simulink model "untitled_restored_from_autosave"  (R2020a)
settings: Solver=VariableStepAuto  StartTime=0.0  StopTime=0.0  RelTol=1e-3
(part 1 of 2)
settings Model: Creator=KevinChan  LastModifiedBy=KevinChan

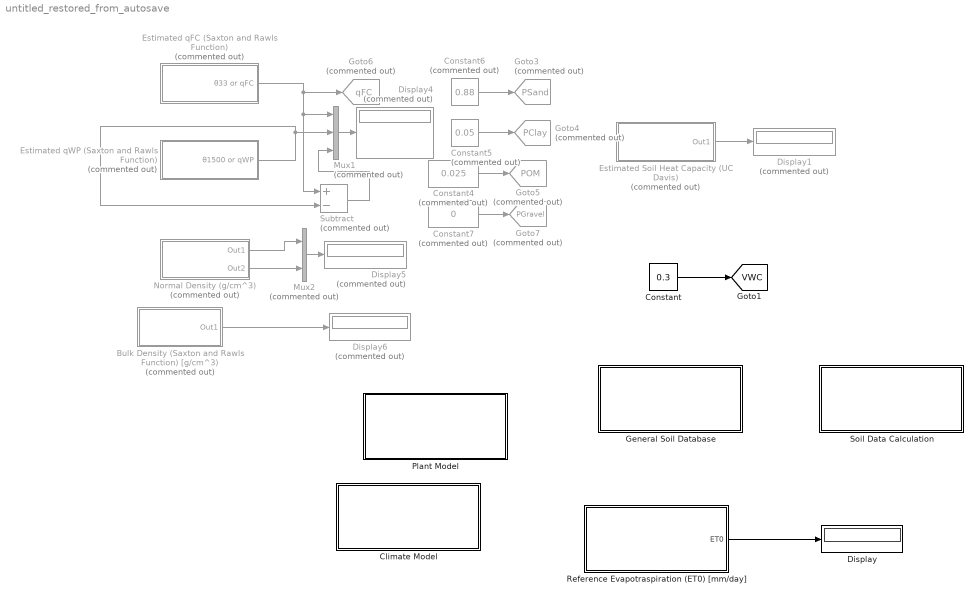
== system untitled_restored_from_autosave ==
  Bulk Density (Saxton and Rawls Function) [g/cm^3) : Subsystem  Commented=on
  Climate Model : Subsystem
  Constant : Constant  Value=0.3
  Constant4 : Constant  Commented=on  Value=0.025
  Constant5 : Constant  Commented=on  Value=0.05
  Constant6 : Constant  Commented=on  Value=0.88
  Constant7 : Constant  Commented=on  Value=0
  Display : Display
  Display{1,4..6} (4 alike) : Display  Commented=on
  Estimated Soil Heat Capacity (UC Davis) : Subsystem  Commented=on
  Estimated qFC (Saxton and Rawls Function) : Subsystem  Commented=on
  Estimated qWP (Saxton and Rawls Function) : Subsystem  Commented=on
  General Soil Database : Subsystem  mask{PGravel=5, PSand=25, PClay=30, POM=5, SM_choice=Estimated Soil Moisture Value, qFC_measured=0, qWP_measured=0, Ze_choice=Estimated, Ze_measured=0}
      mask prompts: PGravel "Percentage of Gravel"; PSand "Percentage of Sand"; PClay "Percentage of Clay"; POM "Percentage of Organic Matter (3-6% if unkown)"; SM_choice "Estimated or measured?"; qFC_measured "Field Capacity Soil Moisture (% Volume in m)"; qWP_measured "Wiliting Point Soil Moisture (% Volume in m)"; Ze_choice "Ze estimated or measured?"; Ze_measured "Enter Ze measured if selected"
      mask TypeOptions SM_choice: Estimated Soil Moisture Value | Measured Soil Moisture Value
      mask TypeOptions Ze_choice: Estimated | Measured
      mask DialogControl Container5 Prompt: Percentage of Gravel (%)
      mask DialogControl ParameterGroupVar Prompt: Percentage of Soil Content excluding Gravel (%)
      mask DialogControl Control2 Prompt: Percentage of Silt is not required
      mask DialogControl Container3 Prompt: Soil Moisture Data (more accurate if measured)
      mask DialogControl Control3 Prompt: Fill the following if you selected measured
      mask DialogControl Container8 Prompt: Ze depth of the surface soil layer that is subject to drying by way of evaporation [0.10-0.15m]
  Goto3 : Goto  Commented=on  GotoTag=PSand  TagVisibility=global
  Goto4 : Goto  Commented=on  GotoTag=PClay  TagVisibility=global
  Goto5 : Goto  Commented=on  GotoTag=POM  TagVisibility=global
  Goto6 : Goto  Commented=on  GotoTag=qFC  TagVisibility=global
  Goto7 : Goto  Commented=on  GotoTag=PGravel  TagVisibility=global
  Mux1 : Mux  Commented=on  Inputs=3
  Mux2 : Mux  Commented=on  Inputs=2
  Normal Density (g/cm^3) : Subsystem  Commented=on
  Plant Model : Subsystem
  Reference Evapotraspiration (ET0) [mm/day] : Subsystem
  Soil Data Calculation : Subsystem
  Subtract : Sum  Commented=on  Inputs=+-
  tag scope: VWC=global
  wires:
  Estimated qFC (Saxton and Rawls Function)/1(" θ33 or qFC") -> Subtract/1, Mux1/1, Goto6/1
  Constant4/1 -> Goto5/1
  Constant5/1 -> Goto4/1
  Constant6/1 -> Goto3/1
  Estimated qWP (Saxton and Rawls Function)/1(θ1500 or qWP) -> Subtract/2, Mux1/2
  Mux1/1 -> Display4/1
  Normal Density (g/cm^3)/1(Out1) -> Mux2/1
  Normal Density (g/cm^3)/2(Out2) -> Mux2/2
  Mux2/1 -> Display5/1
  Bulk Density (Saxton and Rawls Function) [g/cm^3)/1(Out1) -> Display6/1
  Constant7/1 -> Goto7/1
  Reference Evapotraspiration (ET0) [mm/day]/1(ET0) -> Display/1
  Estimated Soil Heat Capacity (UC Davis)/1(Out1) -> Display1/1
  Subtract/1 -> Mux1/3
  Constant/1 -> [VWC]

== system untitled_restored_from_autosave/Bulk Density (Saxton and Rawls Function) [g//cm^3) ==
  Add : Sum
  Constant : Constant
  Constant1 : Constant  Value=2.65
  Normal Density (g/cm^3) : Subsystem
  Product : Product
  Product1 : Product
  Subtract : Sum  Inputs=+-
  Volum Fraction of Gravel (g/cm^3) : Subsystem
  Out1 : Outport
  wires:
  Add/1 -> Out1/1
  Normal Density (g/cm^3)/1(Out1) -> Product/1, Volum Fraction of Gravel (g/cm^3)/1(In1)
  Subtract/1 -> Product/2
  Product/1 -> Add/1
  Constant/1 -> Subtract/1
  Product1/1 -> Add/2
  Constant1/1 -> Product1/2
  Volum Fraction of Gravel (g/cm^3)/1(Out1) -> Subtract/2, Product1/1

== system untitled_restored_from_autosave/Climate Model ==
  " Final Calculation for Data" : Subsystem
  " Historic Data" : Subsystem
  AI Prediction : Subsystem
  General Climate Database : Subsystem  mask{LatDeg=37, LatMin=28, Altitude=9.1, WindH=10}
      mask prompts: LatDeg "Latitude Degree"; LatMin "Latitude Minute"; Altitude "Altitude above Sea Level [m]"; WindH "Height of measurement above ground surface [m]"
      mask DialogControl ParameterGroupVar Prompt: Location
      mask DialogControl Container3 Prompt: Wind Measurement

== system untitled_restored_from_autosave/Estimated Soil Heat Capacity (UC Davis) ==
  Add : Sum
  Bulk Density (Saxton and Rawls Function) [g/cm^3) : Subsystem
  Constant : Constant  Value=837
  Constant1 : Constant  Value=4.19*10^6
  Gain : Gain  Gain=0.001
  Product : Product
  Product1 : Product
  Out1 : Outport
  wires:
  Add/1 -> Out1/1
  Constant/1 -> Product/1
  Bulk Density (Saxton and Rawls Function) [g/cm^3)/1(Out1) -> Gain/1
  Product/1 -> Add/1
  Product1/1 -> Add/2
  Constant1/1 -> Product1/1
  [VWC] -> Product1/2
  Gain/1 -> Product/2

== system untitled_restored_from_autosave/Estimated qFC (Saxton and Rawls Function) ==
  Constant : Constant  Value=1.283
  Constant1 : Constant  Value=0.015
  Constant2 : Constant  Value=0.374
  Product : Product  Inputs=3
  Product1 : Product
  Subtract : Sum  Inputs=++--
  θ33t : Subsystem
  " θ33 or qFC" : Outport
  wires:
  θ33t/1(Out1) -> Product1/1, Product/2, Product/1, Subtract/1
  Product/1 -> Subtract/2
  Constant/1 -> Product/3
  Constant1/1 -> Subtract/4
  Subtract/1 -> " θ33 or qFC"/1
  Product1/1 -> Subtract/3
  Constant2/1 -> Product1/2

== system untitled_restored_from_autosave/Estimated qWP (Saxton and Rawls Function) ==
  Constant : Constant  Value=0.14
  Constant1 : Constant  Value=0.02
  Product : Product
  Subtract : Sum  Inputs=++-
  θ1500t : Subsystem
  θ1500 or qWP : Outport
  wires:
  Subtract/1 -> θ1500 or qWP/1
  Constant/1 -> Product/2
  θ1500t/1(Out1) -> Subtract/1, Product/1
  Constant1/1 -> Subtract/3
  Product/1 -> Subtract/2

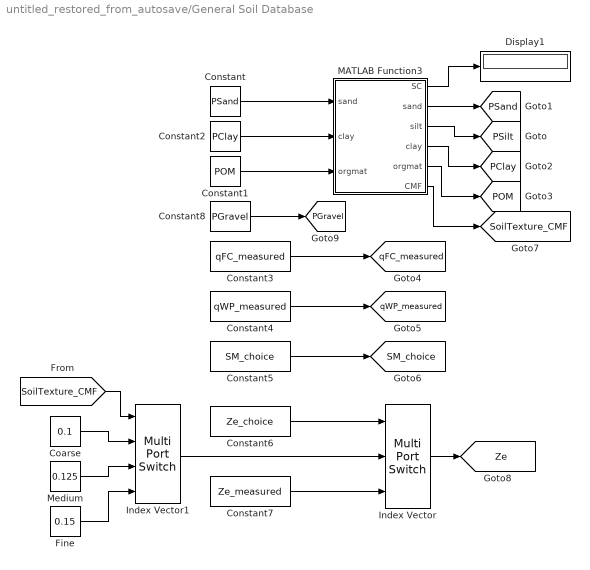
== system untitled_restored_from_autosave/General Soil Database ==
  Coarse : Constant  Value=0.1
  Constant : Constant  Value=PSand
  Constant1 : Constant  Value=POM
  Constant2 : Constant  Value=PClay
  Constant3 : Constant  Value=qFC_measured
  Constant4 : Constant  Value=qWP_measured
  Constant5 : Constant  Value=SM_choice
  Constant6 : Constant  Value=Ze_choice
  Constant7 : Constant  Value=Ze_measured
  Constant8 : Constant  Value=PGravel
  Display1 : Display
  Fine : Constant  Value=0.15
  Index Vector : MultiPortSwitch  Inputs=2
  Index Vector1 : MultiPortSwitch
  MATLAB Function3 : MATLAB Function  TreatAsAtomicUnit=on
  Medium : Constant  Value=0.125
  tag scope: PClay=global, PGravel=global, POM=global, PSand=global, PSilt=global, SM_choice=global, SoilTexture_CMF=global, Ze=global, qFC_measured=global, qWP_measured=global
  wires:
  MATLAB Function3/1(SC) -> Display1/1
  Constant2/1 -> MATLAB Function3/2("clay ")
  Constant1/1 -> MATLAB Function3/3("orgmat ")
  Constant/1 -> MATLAB Function3/1("sand ")
  MATLAB Function3/3(silt) -> [PSilt]
  Constant3/1 -> [qFC_measured]
  Constant4/1 -> [qWP_measured]
  Constant5/1 -> [SM_choice]
  MATLAB Function3/5(orgmat) -> [POM]
  MATLAB Function3/2(sand) -> [PSand]
  MATLAB Function3/4(clay) -> [PClay]
  MATLAB Function3/6(CMF) -> [SoilTexture_CMF]
  Constant6/1 -> Index Vector/1
  Constant7/1 -> Index Vector/3
  [SoilTexture_CMF] -> Index Vector1/1
  Index Vector1/1 -> Index Vector/2
  Coarse/1 -> Index Vector1/2
  Fine/1 -> Index Vector1/4
  Medium/1 -> Index Vector1/3
  Index Vector/1 -> [Ze]
  Constant8/1 -> [PGravel]

== system untitled_restored_from_autosave/Normal Density (g//cm^3) ==
  Constant : Constant  Value=2.65
  Constant1 : Constant
  Product : Product
  Saturated Moisture θS : Subsystem
  Subtract : Sum  Inputs=+-
  Out1 : Outport
  Out2 : Outport  Port=2
  wires:
  Product/1 -> Out1/1
  Constant/1 -> Product/2
  Subtract/1 -> Product/1
  Constant1/1 -> Subtract/1
  Saturated Moisture θS/1(Out1) -> Out2/1, Subtract/2

== system untitled_restored_from_autosave/Plant Model ==
  General Plant Database : Subsystem  mask{CropName=Maize, PD_Year=2020, PD_Month=11, PD_Day=28, Lini=0, Ldev=0, Lmid=0, Llate=0, inf_depth=0, interval_irr=1 day, Kc_ini=0, Kc_mid=0, Kc_end=0, MaxCropH=0, Kcb_ini=0, Kcb_mid=0, Kcb_end=0}
      mask prompts: CropName "Crop Name"; PD_Year "Year"; PD_Month "Month"; PD_Day "Day"; Lini "Initial Stage"; Ldev "Devloping Stage"; Lmid "Mid-season Stage"; Llate "Late Season Stage"; inf_depth "Average infiltration depth [mm]."; interval_irr "Interval of Irrigation (0 if unkwon)"; Kc_ini "Enter Kc ini from the Table"; Kc_mid "Enter Kc mid from the Table"; Kc_end "Enter Kc end from the Table"; MaxCropH "Enter Maximum Crop Height (h) (m) from the Table"; Kcb_ini "Enter Kcb ini from the Table"; Kcb_mid "Enter Kcb mid from the Table"; Kcb_end "Enter Kcb end from the Table"
      mask TypeOptions interval_irr: 1 day | 2 days | 4 days | 7 days | 10 days | 20 days
      mask DialogControl ParameterGroupVar Prompt: General
      mask DialogControl Control2 Prompt: Plant Date:
      mask DialogControl Container3 Prompt: Lengths of Crop Develop Stages
      mask DialogControl Control3 Prompt: Find the values in the following link with corresponding crop type and closest plant date:
      mask DialogControl Control4 Prompt: http://www.fao.org/3/x0490e/x0490e0b.htm#length%20of%20growth%20stages
      mask DialogControl Container4 Prompt: Single Crop Coefficients
      mask DialogControl Control5 Prompt: Find the values for your corresponding crop in the following table:
      mask DialogControl Control6 Prompt: http://www.fao.org/3/x0490e/x0490e0b.htm#tabulated%20kc%20values
      mask DialogControl Container5 Prompt: Dual Crop Coefficents
      mask DialogControl Control7 Prompt: Find the values for your corresponding crop in the following table:
      mask DialogControl Control8 Prompt: http://www.fao.org/3/x0490e/x0490e0c.htm#basal%20crop%20coefficient%20(kcb)
  Plant Data Calculation : Subsystem

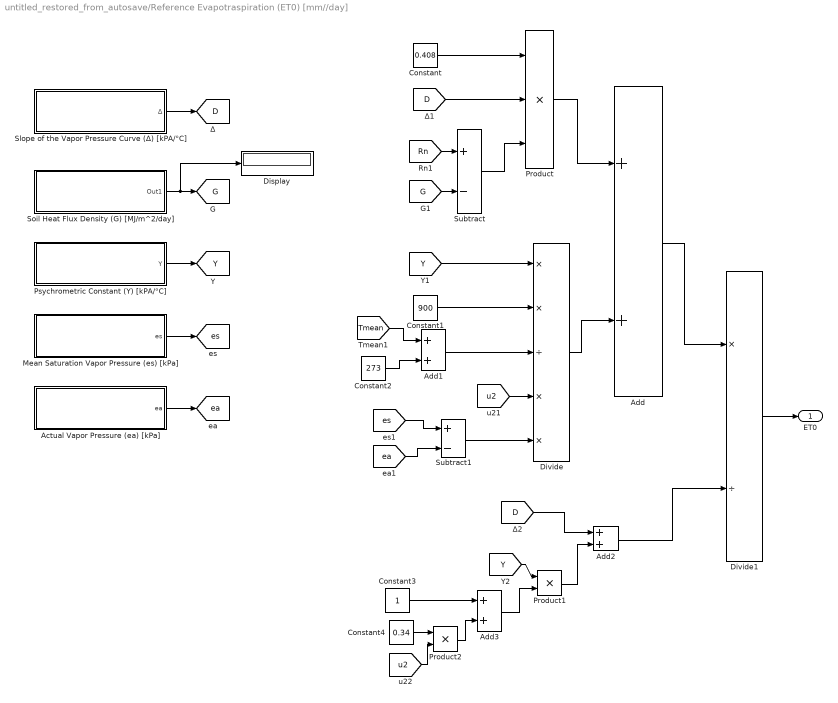
== system untitled_restored_from_autosave/Reference Evapotraspiration (ET0) [mm//day] ==
  Actual Vapor Pressure (ea) [kPa] : Subsystem  mask{ea_choice=Derived from Dewpoint Temperature, apsy_choice=0.000662 for ventilated (Asmann type) psychrometers, with an air movement of some 5 m/s}
      mask prompts: ea_choice "Select which method to derive:"; apsy_choice "Pick value for apsy:"
      mask init:
      | apsy = 0;
      | 
      | if apsy_choice == 1
      |     apsy = 0.000662;
      | elseif apsy_choice == 2
      |     apsy = 0.000800;
      | elseif apsy_choice == 3
      |     apsy = 0.001200;
      | end
      mask TypeOptions ea_choice: Derived from Dewpoint Temperature | Derived from Psyschrometirc Data | Derived from Relative Humidity Data (RHmax and RHmin) | Derived from Relative Humidity Data (RHmax only) | Derived from Relative Humidity Data (RHmean only)
      mask TypeOptions apsy_choice: 0.000662 for ventilated (Asmann type) psychrometers, with an air movement of some 5 m/s | 0.000800 for natural ventilated psychrometers (about 1 m/s) | 0.001200 for non-ventilated psychrometers installed indoors.
      mask DialogControl Control2 Prompt: There are 3 different ways to derive the actual vapor pressure. Depend on what data you have avaliable, pick the following choices. If you are picking relatitive humidity, beware of the following. When using equipment where errors in estimating RHmin can be large, or when RH data integrity are in doubt, then one should use only RHmax. In the absence of RHmax and RHmin, you can select to use RHmean.
      mask DialogControl Control3 Prompt: If you picked to use Psychrometric Data, select the folowing.
  Add{,1..3} (4 alike) : Sum
  Constant : Constant  Value=0.408
  Constant1 : Constant  Value=900
  Constant2 : Constant  Value=273
  Constant3 : Constant
  Constant4 : Constant  Value=0.34
  Display : Display
  Divide : Product  Inputs=**/**
  Divide1 : Product  Inputs=*/
  "Mean Saturation Vapor Pressure (es) [kPa] " : Subsystem
  Product : Product  Inputs=3
  Product1 : Product
  Product2 : Product
  Psychrometric Constant (Y) [kPA/°C] : Subsystem
  Slope of the Vapor Pressure Curve (∆) [kPA/°C] : Subsystem
  Soil Heat Flux Density (G) [MJ/m^2/day] : Subsystem  mask{G_choice=For day and ten-day periods}
      mask prompts: G_choice "Select Time Step:"
      mask TypeOptions G_choice: For day and ten-day periods | For long periods
      mask DialogControl Control2 Prompt: For daily or weekly periods of time, soil heat flux density is small and can be ignored. A method to find G for long period of time is here, based on the idea that the soil temperature follows air temperature.
  Subtract : Sum  Inputs=+-
  Subtract1 : Sum  Inputs=+-
  ET0 : Outport
  tag scope: D=global, G=global, Y=global, ea=global, es=global
  wires:
  Divide1/1 -> ET0/1
  Constant/1 -> Product/1
  [D] -> Product/2
  [Rn] -> Subtract/1
  [G] -> Subtract/2
  Subtract/1 -> Product/3
  Product/1 -> Add/1
  Divide/1 -> Add/2
  Constant1/1 -> Divide/2
  [Tmean] -> Add1/1
  Constant2/1 -> Add1/2
  Add1/1 -> Divide/3
  Subtract1/1 -> Divide/5
  [es] -> Subtract1/1
  [ea] -> Subtract1/2
  Add/1 -> Divide1/1
  Add2/1 -> Divide1/2
  Product1/1 -> Add2/2
  Add3/1 -> Product1/2
  Constant3/1 -> Add3/1
  Product2/1 -> Add3/2
  Slope of the Vapor Pressure Curve (∆) [kPA/°C]/1(∆) -> [D]
  [D] -> Add2/1
  Soil Heat Flux Density (G) [MJ/m^2/day]/1(Out1) -> Display/1, [G]
  Psychrometric Constant (Y) [kPA/°C]/1(Y) -> [Y]
  [Y] -> Divide/1
  [Y] -> Product1/1
  [u2] -> Divide/4
  [u2] -> Product2/2
  "Mean Saturation Vapor Pressure (es) [kPa] "/1(es) -> [es]
  Actual Vapor Pressure (ea) [kPa]/1(ea) -> [ea]
  Constant4/1 -> Product2/1

== system untitled_restored_from_autosave/Soil Data Calculation ==
  Demux : Demux  Outputs=2
  Display : Display
  Estimated Soil Heat Capacity (UC Davis) : Subsystem
  Estimated qFC (Saxton and Rawls Function) : Subsystem
  Estimated qWP (Saxton and Rawls Function) : Subsystem
  Gain : Gain  Gain=10^(-6)
  Index Vector : MultiPortSwitch  Inputs=2
  Mux : Mux  Inputs=2
  Mux1 : Mux  Inputs=2
  tag scope: cs=global, qFC=global, qWP=global
  wires:
  [SM_choice] -> Index Vector/1
  [qFC_measured] -> Mux/1
  [qWP_measured] -> Mux/2
  Mux/1 -> Index Vector/3
  Index Vector/1 -> Demux/1
  Demux/1 -> [qFC]
  Demux/2 -> [qWP]
  Mux1/1 -> Index Vector/2
  Estimated qFC (Saxton and Rawls Function)/1(" θ33 or qFC") -> Mux1/1
  Estimated qWP (Saxton and Rawls Function)/1(θ1500 or qWP) -> Mux1/2
  Estimated Soil Heat Capacity (UC Davis)/1(Out1) -> Gain/1
  Gain/1 -> Display/1, [cs]

== system untitled_restored_from_autosave/Bulk Density (Saxton and Rawls Function) [g//cm^3)/Normal Density (g//cm^3) ==
  Constant : Constant  Value=2.65
  Constant1 : Constant
  Product : Product
  Saturated Moisture θS : Subsystem
  Subtract : Sum  Inputs=+-
  Out1 : Outport
  wires:
  Product/1 -> Out1/1
  Constant/1 -> Product/2
  Subtract/1 -> Product/1
  Constant1/1 -> Subtract/1
  Saturated Moisture θS/1(Out1) -> Subtract/2

== system untitled_restored_from_autosave/Bulk Density (Saxton and Rawls Function) [g//cm^3)/Volum Fraction of Gravel (g//cm^3) ==
  In1 : Inport
  Constant : Constant  Value=2.65
  Constant1 : Constant
  Constant2 : Constant
  Divide : Product  Inputs=*/
  Divide1 : Product  Inputs=*/
  Product : Product
  Product1 : Product
  Subtract : Sum  Inputs=+-
  Subtract1 : Sum  Inputs=+-
  Out1 : Outport
  wires:
  In1/1 -> Divide/1
  [PGravel] -> Product1/1, Product/2
  Constant/1 -> Divide/2
  Divide/1 -> Subtract1/2, Product/1
  Product/1 -> Divide1/1
  Subtract/1 -> Divide1/2
  Constant1/1 -> Subtract/1
  Product1/1 -> Subtract/2
  Subtract1/1 -> Product1/2
  Constant2/1 -> Subtract1/1
  Divide1/1 -> Out1/1

== system untitled_restored_from_autosave/Climate Model/ Final Calculation for Data ==
  Atmospheric Pressure [kPa] : Subsystem
  Constant : Constant  Value=101.8
  Daily Temperature [°C] : Subsystem
  Display : Display
  Humidity : Subsystem
  Net Radiation at the Crop Surface (Rn) [MJ/m^2/day] : Subsystem
  Precipitation : Subsystem
  Wind Speed : Subsystem
  tag scope: P=global, RHmax=global, RHmean=global, RHmin=global, Rn=global, Tdew=global, Tdry=global, Tmax=global, Tmean=global, Tmin=global, Tpast=global, Tpast_t=global, Twet=global, u2=global
  wires:
  Daily Temperature [°C]/1(Tmax) -> [Tmax]
  Daily Temperature [°C]/2(Tmin) -> [Tmin]
  Daily Temperature [°C]/3(Tmean) -> [Tmean]
  Net Radiation at the Crop Surface (Rn) [MJ/m^2/day]/1(Rn) -> [Rn]
  Wind Speed/1(Out1) -> [u2]
  Daily Temperature [°C]/4(Tdew) -> [Tdew]
  Daily Temperature [°C]/5(Tdry) -> [Tdry]
  Daily Temperature [°C]/6(Twet) -> [Twet]
  Humidity/1(RHmax) -> [RHmax]
  Humidity/3(RHmean) -> [RHmean]
  Humidity/2(RHmin) -> [RHmin]
  Daily Temperature [°C]/7(Tpast) -> [Tpast]
  Daily Temperature [°C]/8(Tpast_time) -> [Tpast_t]
  Constant/1 -> [P]
  Atmospheric Pressure [kPa]/1(P) -> Display/1

== system untitled_restored_from_autosave/Climate Model/ Historic Data ==
  Humidity : Subsystem
  Precipitation : Subsystem
  Solar Radiation : Subsystem
  Temperature [°C] : Subsystem
  "Wind Speed " : Subsystem

== system untitled_restored_from_autosave/Climate Model/AI Prediction ==
  AI Solar Radiation [MJ/m^2/day] : Subsystem
  Humidity : Subsystem
  Precipitation : Subsystem
  Temperature [°C] : Subsystem
  Wind Speed [m/s] : Subsystem
  tag scope: AI_Rs=global, AI_T=global, AI_Uz=global
  wires:
  AI Solar Radiation [MJ/m^2/day]/1(AI_Rs) -> [AI_Rs]
  Wind Speed [m/s]/1(AI_Uz) -> [AI_Uz]
  Temperature [°C]/1(AI_T) -> [AI_T]

== system untitled_restored_from_autosave/Climate Model/General Climate Database ==
  Altitude : Constant  Value=Altitude
  LatDeg : Constant  Value=LatDeg
  LatMin : Constant  Value=LatMin
  WindH : Constant  Value=WindH
  tag scope: Altitude=global, LatDeg=global, LatMin=global, WindH=global
  wires:
  Altitude/1 -> [Altitude]
  LatDeg/1 -> [LatDeg]
  LatMin/1 -> [LatMin]
  WindH/1 -> [WindH]

== system untitled_restored_from_autosave/Estimated Soil Heat Capacity (UC Davis)/Bulk Density (Saxton and Rawls Function) [g//cm^3) ==
  Add : Sum
  Constant : Constant
  Constant1 : Constant  Value=2.65
  Normal Density (g/cm^3) : Subsystem
  Product : Product
  Product1 : Product
  Subtract : Sum  Inputs=+-
  Volum Fraction of Gravel (g/cm^3) : Subsystem
  Out1 : Outport
  wires:
  Add/1 -> Out1/1
  Normal Density (g/cm^3)/1(Out1) -> Product/1, Volum Fraction of Gravel (g/cm^3)/1(In1)
  Subtract/1 -> Product/2
  Product/1 -> Add/1
  Constant/1 -> Subtract/1
  Product1/1 -> Add/2
  Constant1/1 -> Product1/2
  Volum Fraction of Gravel (g/cm^3)/1(Out1) -> Subtract/2, Product1/1

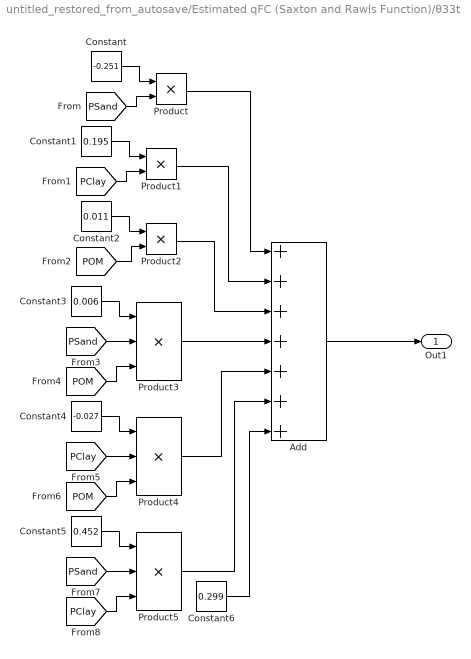
== system untitled_restored_from_autosave/Estimated qFC (Saxton and Rawls Function)/θ33t ==
  Add : Sum  Inputs=+++++++
  Constant : Constant  Value=-0.251
  Constant1 : Constant  Value=0.195
  Constant2 : Constant  Value=0.011
  Constant3 : Constant  Value=0.006
  Constant4 : Constant  Value=-0.027
  Constant5 : Constant  Value=0.452
  Constant6 : Constant  Value=0.299
  Product : Product
  Product1 : Product
  Product2 : Product
  Product3 : Product  Inputs=3
  Product4 : Product  Inputs=3
  Product5 : Product  Inputs=3
  Out1 : Outport
  wires:
  [PClay] -> Product5/3
  [PClay] -> Product1/2
  Constant4/1 -> Product4/1
  Product1/1 -> Add/2
  Constant3/1 -> Product3/1
  Product5/1 -> Add/6
  [PClay] -> Product4/2
  Product4/1 -> Add/5
  Constant6/1 -> Add/7
  Constant5/1 -> Product5/1
  [PSand] -> Product5/2
  Product/1 -> Add/1
  [PSand] -> Product/2
  Product2/1 -> Add/3
  Constant2/1 -> Product2/1
  Constant1/1 -> Product1/1
  Product3/1 -> Add/4
  Constant/1 -> Product/1
  [POM] -> Product2/2
  [PSand] -> Product3/2
  [POM] -> Product4/3
  [POM] -> Product3/3
  Add/1 -> Out1/1

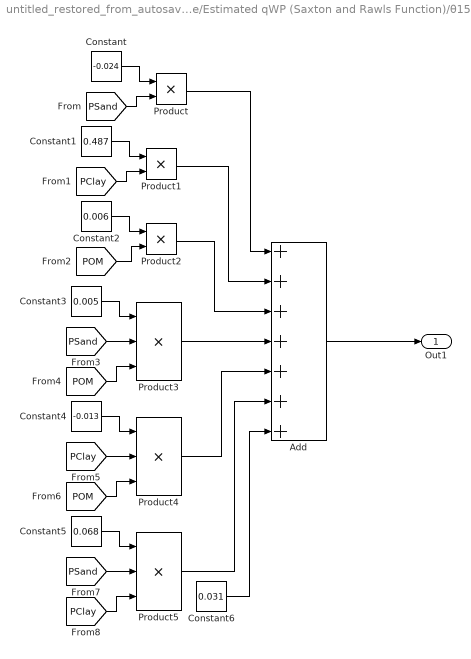
== system untitled_restored_from_autosave/Estimated qWP (Saxton and Rawls Function)/θ1500t ==
  Add : Sum  Inputs=+++++++
  Constant : Constant  Value=-0.024
  Constant1 : Constant  Value=0.487
  Constant2 : Constant  Value=0.006
  Constant3 : Constant  Value=0.005
  Constant4 : Constant  Value=-0.013
  Constant5 : Constant  Value=0.068
  Constant6 : Constant  Value=0.031
  Product : Product
  Product1 : Product
  Product2 : Product
  Product3 : Product  Inputs=3
  Product4 : Product  Inputs=3
  Product5 : Product  Inputs=3
  Out1 : Outport
  wires:
  [PClay] -> Product5/3
  [PClay] -> Product1/2
  Constant4/1 -> Product4/1
  Product1/1 -> Add/2
  Constant3/1 -> Product3/1
  Product5/1 -> Add/6
  [PClay] -> Product4/2
  Product4/1 -> Add/5
  Constant6/1 -> Add/7
  Constant5/1 -> Product5/1
  [PSand] -> Product5/2
  Product/1 -> Add/1
  [PSand] -> Product/2
  Product2/1 -> Add/3
  Constant2/1 -> Product2/1
  Constant1/1 -> Product1/1
  Product3/1 -> Add/4
  Constant/1 -> Product/1
  [POM] -> Product2/2
  [PSand] -> Product3/2
  [POM] -> Product4/3
  [POM] -> Product3/3
  Add/1 -> Out1/1

== system untitled_restored_from_autosave/Normal Density (g//cm^3)/Saturated Moisture θS ==
  Constant : Constant  Value=0.097
  Constant1 : Constant  Value=0.043
  Product : Product
  Subtract : Sum  Inputs=++-+
  θ(S-33) : Subsystem
  Out1 : Outport
  wires:
  Subtract/1 -> Out1/1
  [qFC] -> Subtract/1
  Product/1 -> Subtract/3
  Constant/1 -> Product/1
  [PSand] -> Product/2
  Constant1/1 -> Subtract/4
  θ(S-33)/1(Out1) -> Subtract/2

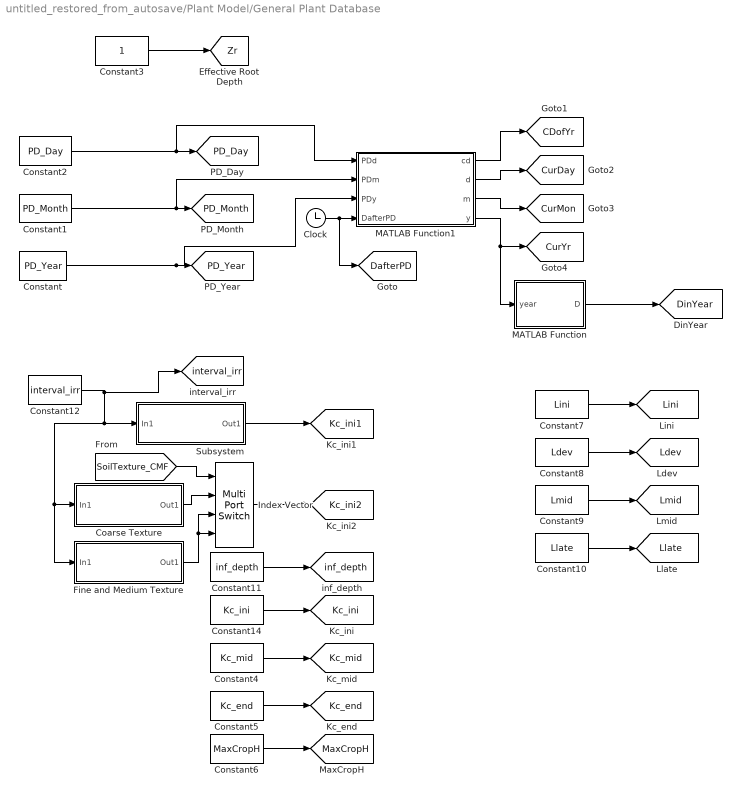
== system untitled_restored_from_autosave/Plant Model/General Plant Database ==
  Clock : Clock
  Coarse Texture : Subsystem
  Constant : Constant  Value=PD_Year
  Constant1 : Constant  Value=PD_Month
  Constant10 : Constant  Value=Llate
  Constant11 : Constant  Value=inf_depth
  Constant12 : Constant  Value=interval_irr
  Constant14 : Constant  Value=Kc_ini
  Constant2 : Constant  Value=PD_Day
  Constant3 : Constant
  Constant4 : Constant  Value=Kc_mid
  Constant5 : Constant  Value=Kc_end
  Constant6 : Constant  Value=MaxCropH
  Constant7 : Constant  Value=Lini
  Constant8 : Constant  Value=Ldev
  Constant9 : Constant  Value=Lmid
  Fine and Medium Texture : Subsystem
  Index Vector : MultiPortSwitch
  MATLAB Function : MATLAB Function  TreatAsAtomicUnit=on
  MATLAB Function1 : MATLAB Function  TreatAsAtomicUnit=on
  Subsystem : Subsystem
  tag scope: CDofYr=global, CurDay=global, CurMon=global, CurYr=global, DafterPD=global, DinYear=global, Kc_end=global, Kc_ini1=global, Kc_ini2=global, Kc_ini=global, Kc_mid=global, Ldev=global, Lini=global, Llate=global, Lmid=global, MaxCropH=global, PD_Day=global, PD_Month=global, PD_Year=global, Zr=global, inf_depth=global, interval_irr=global
  wires:
  Constant/1 -> MATLAB Function1/3(PDy), [PD_Year]
  Constant1/1 -> MATLAB Function1/2(PDm), [PD_Month]
  Constant2/1 -> MATLAB Function1/1(PDd), [PD_Day]
  MATLAB Function/1(D) -> [DinYear]
  Constant4/1 -> [Kc_mid]
  Constant5/1 -> [Kc_end]
  Constant6/1 -> [MaxCropH]
  Constant9/1 -> [Lmid]
  Constant8/1 -> [Ldev]
  Constant7/1 -> [Lini]
  Constant10/1 -> [Llate]
  Constant11/1 -> [inf_depth]
  [SoilTexture_CMF] -> Index Vector/1
  Index Vector/1 -> [Kc_ini2]
  Constant12/1 -> [interval_irr], Fine and Medium Texture/1(In1), Coarse Texture/1(In1), Subsystem/1(In1)
  Subsystem/1(Out1) -> [Kc_ini1]
  Coarse Texture/1(Out1) -> Index Vector/2
  Constant14/1 -> [Kc_ini]
  Clock/1 -> MATLAB Function1/4(DafterPD), [DafterPD]
  MATLAB Function1/1(cd) -> [CDofYr]
  MATLAB Function1/2(d) -> [CurDay]
  MATLAB Function1/3(m) -> [CurMon]
  MATLAB Function1/4(y) -> MATLAB Function/1(year), [CurYr]
  Fine and Medium Texture/1(Out1) -> Index Vector/3, Index Vector/4
  Constant3/1 -> [Zr]

== system untitled_restored_from_autosave/Plant Model/Plant Data Calculation ==
  MATLAB Function : MATLAB Function  TreatAsAtomicUnit=on
  tag scope: Ps=global
  wires:
  MATLAB Function/1(stage) -> [Ps]
  [DafterPD] -> MATLAB Function/1(d)
  [Lini] -> MATLAB Function/2(Lini)
  [Ldev] -> MATLAB Function/3(Ldev)
  [Lmid] -> MATLAB Function/4(Lmid)
  [Llate] -> MATLAB Function/5(Llate)

== system untitled_restored_from_autosave/Reference Evapotraspiration (ET0) [mm//day]/Actual Vapor Pressure (ea) [kPa] ==
  Constant : Constant  Value=ea_choice
  Derived from Dewpoint Temperature : Subsystem
  Derived from Psychrometric Data : Subsystem
  Derived from RHmax & RHmin : Subsystem
  Derived from RHmax only : Subsystem
  Derived from RHmean only : Subsystem
  Index Vector : MultiPortSwitch  Inputs=5
  ea : Outport
  wires:
  Derived from Dewpoint Temperature/1(Out1) -> Index Vector/2
  Index Vector/1 -> ea/1
  Constant/1 -> Index Vector/1
  Derived from Psychrometric Data/1(Out1) -> Index Vector/3
  Derived from RHmean only/1(Out1) -> Index Vector/6
  Derived from RHmax only/1(Out1) -> Index Vector/5
  Derived from RHmax & RHmin/1(Out1) -> Index Vector/4

== system untitled_restored_from_autosave/Reference Evapotraspiration (ET0) [mm//day]/Mean Saturation Vapor Pressure (es) [kPa]  ==
  Add2 : Sum
  Constant6 : Constant  Value=2
  Divide2 : Product  Inputs=*/
  Saturation Vapor Pressure (eo) : Subsystem
  Saturation Vapor Pressure (eo) 2 : Subsystem
  es : Outport
  wires:
  Add2/1 -> Divide2/1
  Divide2/1 -> es/1
  Constant6/1 -> Divide2/2
  [Tmax] -> Saturation Vapor Pressure (eo)/1(In1)
  Saturation Vapor Pressure (eo)/1(Out1) -> Add2/1
  [Tmin] -> Saturation Vapor Pressure (eo) 2/1(In1)
  Saturation Vapor Pressure (eo) 2/1(Out1) -> Add2/2

== system untitled_restored_from_autosave/Reference Evapotraspiration (ET0) [mm//day]/Psychrometric Constant (Y) [kPA//°C] ==
  Divide : Product  Inputs=**//
  Latent Heat of Vaporization (l) [MJ/kg] : Subsystem
  Ratio Molecular Weight of Water Vapour/Dry Air (e) : Constant  Value=0.622
  "Specific Heat at Constant Pressure (cp) [MJ/kg/°C] " : Constant  Value=0.001013
  Y : Outport
  wires:
  Divide/1 -> Y/1
  "Specific Heat at Constant Pressure (cp) [MJ/kg/°C] "/1 -> Divide/1
  Latent Heat of Vaporization (l) [MJ/kg]/1(l) -> Divide/4
  [P] -> Divide/2
  Ratio Molecular Weight of Water Vapour/Dry Air (e)/1 -> Divide/3

== system untitled_restored_from_autosave/Reference Evapotraspiration (ET0) [mm//day]/Slope of the Vapor Pressure Curve (∆) [kPA//°C] ==
  Add : Sum
  Constant : Constant  Value=4098
  Constant1 : Constant  Value=0.6108
  Constant2 : Constant  Value=17.27
  Constant3 : Constant  Value=237.3
  Divide : Product  Inputs=***//
  Divide1 : Product  Inputs=**/
  Math Function : Math  SaturateOnIntegerOverflow=on
  ∆ : Outport
  wires:
  Divide/1 -> ∆/1
  Constant/1 -> Divide/1
  Constant1/1 -> Divide/2
  Math Function/1 -> Divide/3
  Divide1/1 -> Math Function/1
  [Tmean] -> Add/1, Divide1/2
  Constant2/1 -> Divide1/1
  Add/1 -> Divide/5, Divide/4, Divide1/3
  Constant3/1 -> Add/2

== system untitled_restored_from_autosave/Reference Evapotraspiration (ET0) [mm//day]/Soil Heat Flux Density (G) [MJ//m^2//day] ==
  Constant : Constant  Value=G_choice
  For day and ten-day peroids : Constant  Value=0
  Index Vector : MultiPortSwitch  Inputs=2
  Long Time Steps : Subsystem
  Out1 : Outport
  wires:
  Long Time Steps/1(Out1) -> Index Vector/3
  For day and ten-day peroids/1 -> Index Vector/2
  Constant/1 -> Index Vector/1
  Index Vector/1 -> Out1/1

== system untitled_restored_from_autosave/Soil Data Calculation/Estimated Soil Heat Capacity (UC Davis) ==
  Add : Sum
  Bulk Density (Saxton and Rawls Function) [g/cm^3) : Subsystem
  Constant : Constant  Value=837
  Constant1 : Constant  Value=4.19*10^6
  Gain : Gain  Gain=0.001
  Product : Product
  Product1 : Product
  Out1 : Outport
  wires:
  Add/1 -> Out1/1
  Constant/1 -> Product/1
  Bulk Density (Saxton and Rawls Function) [g/cm^3)/1(Out1) -> Gain/1
  Product/1 -> Add/1
  Product1/1 -> Add/2
  Constant1/1 -> Product1/1
  [VWC] -> Product1/2
  Gain/1 -> Product/2

== system untitled_restored_from_autosave/Soil Data Calculation/Estimated qFC (Saxton and Rawls Function) ==
  Constant : Constant  Value=1.283
  Constant1 : Constant  Value=0.015
  Constant2 : Constant  Value=0.374
  Product : Product  Inputs=3
  Product1 : Product
  Subtract : Sum  Inputs=++--
  θ33t : Subsystem
  " θ33 or qFC" : Outport
  wires:
  θ33t/1(Out1) -> Product1/1, Product/2, Product/1, Subtract/1
  Product/1 -> Subtract/2
  Constant/1 -> Product/3
  Constant1/1 -> Subtract/4
  Subtract/1 -> " θ33 or qFC"/1
  Product1/1 -> Subtract/3
  Constant2/1 -> Product1/2

== system untitled_restored_from_autosave/Soil Data Calculation/Estimated qWP (Saxton and Rawls Function) ==
  Constant : Constant  Value=0.14
  Constant1 : Constant  Value=0.02
  Product : Product
  Subtract : Sum  Inputs=++-
  θ1500t : Subsystem
  θ1500 or qWP : Outport
  wires:
  Subtract/1 -> θ1500 or qWP/1
  Constant/1 -> Product/2
  θ1500t/1(Out1) -> Subtract/1, Product/1
  Constant1/1 -> Subtract/3
  Product/1 -> Subtract/2

== system untitled_restored_from_autosave/Bulk Density (Saxton and Rawls Function) [g//cm^3)/Normal Density (g//cm^3)/Saturated Moisture θS ==
  Constant : Constant  Value=0.097
  Constant1 : Constant  Value=0.043
  Product : Product
  Subtract : Sum  Inputs=++-+
  θ(S-33) : Subsystem
  Out1 : Outport
  wires:
  Subtract/1 -> Out1/1
  [qFC] -> Subtract/1
  Product/1 -> Subtract/3
  Constant/1 -> Product/1
  [PSand] -> Product/2
  Constant1/1 -> Subtract/4
  θ(S-33)/1(Out1) -> Subtract/2

== system untitled_restored_from_autosave/Climate Model/ Final Calculation for Data/Atmospheric Pressure [kPa] ==
  Constant : Constant  Value=101.3
  Constant1 : Constant  Value=5.26
  Constant2 : Constant  Value=293
  Constant3 : Constant  Value=0.0065
  Constant5 : Constant  Value=293
  Divide : Product  Inputs=*/
  Math Function : Math  Operator=pow  SaturateOnIntegerOverflow=on
  Product : Product
  Product1 : Product
  Subtract : Sum  Inputs=+-
  P : Outport
  wires:
  Product/1 -> P/1
  Constant/1 -> Product/1
  Math Function/1 -> Product/2
  Constant1/1 -> Math Function/2
  Divide/1 -> Math Function/1
  Subtract/1 -> Divide/1
  Constant2/1 -> Subtract/1
  Product1/1 -> Subtract/2
  Constant3/1 -> Product1/1
  [Altitude] -> Product1/2
  Constant5/1 -> Divide/2

== system untitled_restored_from_autosave/Climate Model/ Final Calculation for Data/Daily Temperature [°C] ==
  Constant : Constant  Value=14
  Constant1 : Constant  Value=8.7
  Constant2 : Constant  Value=11.1
  Constant3 : Constant  Value=10
  Constant4 : Constant  Value=10
  Constant5 : Constant
  Mean Air Temperature at 2m height (Tmean) [°C] : Subsystem
  Tmax : Outport
  Tmin : Outport  Port=2
  Tmean : Outport  Port=3
  Tdew : Outport  Port=4
  Tdry : Outport  Port=5
  Twet : Outport  Port=6
  Tpast : Outport  Port=7
  Tpast_time : Outport  Port=8
  wires:
  Mean Air Temperature at 2m height (Tmean) [°C]/1(Out1) -> Tmean/1
  Constant/1 -> Tmax/1
  Constant1/1 -> Tmin/1
  Constant2/1 -> Mean Air Temperature at 2m height (Tmean) [°C]/1(In1)
  Constant3/1 -> Tdew/1
  Constant4/1 -> Tpast/1
  Constant5/1 -> Tpast_time/1

== system untitled_restored_from_autosave/Climate Model/ Final Calculation for Data/Humidity ==
  Constant : Constant  Value=96
  Constant1 : Constant  Value=79
  Constant2 : Constant  Value=92.2
  RHmax : Outport
  RHmin : Outport  Port=2
  RHmean : Outport  Port=3
  wires:
  Constant/1 -> RHmax/1
  Constant1/1 -> RHmin/1
  Constant2/1 -> RHmean/1

== system untitled_restored_from_autosave/Climate Model/ Final Calculation for Data/Net Radiation at the Crop Surface (Rn) [MJ//m^2//day] ==
  Clear-Sky Solar Radiation (Rso) [MJ/m^2/day] : Subsystem
  Extraterrestrial Radiation (Ra) [MJ/m^2/day] : Subsystem
  Net Longwave Radiation (Rnl) [MJ/m^2/day] : Subsystem
  Net Solar/Shortwave Radiation (Rns) [MJ/m^2/day] : Subsystem
  Solar Radiation (Rs) [MJ/m^2/day] : Subsystem  mask{Ac_Rs=AI Predicted Solar Radiation}
      mask prompts: Ac_Rs "How to calculate Solar Radiation? (Most to Least Accurate)"
      mask TypeOptions Ac_Rs: AI Predicted Solar Radiation | Angstrom Formula if AI_Rs not avaliable | Hargreaves Formula if AI_Rs and hour of daylight is not available
  Subtract : Sum  Inputs=+-
  Rn : Outport
  tag scope: Ra=global, Rs=global, Rso=global
  wires:
  Subtract/1 -> Rn/1
  Net Solar/Shortwave Radiation (Rns) [MJ/m^2/day]/1(Out1) -> Subtract/1
  Net Longwave Radiation (Rnl) [MJ/m^2/day]/1(Rnl) -> Subtract/2
  Solar Radiation (Rs) [MJ/m^2/day]/1(Rs) -> [Rs]
  Extraterrestrial Radiation (Ra) [MJ/m^2/day]/1(Ra) -> [Ra]
  [CDofYr] -> Extraterrestrial Radiation (Ra) [MJ/m^2/day]/1(J)
  Clear-Sky Solar Radiation (Rso) [MJ/m^2/day]/1(Rso) -> [Rso]

== system untitled_restored_from_autosave/Climate Model/ Final Calculation for Data/Precipitation ==

== system untitled_restored_from_autosave/Climate Model/ Final Calculation for Data/Wind Speed ==
  Constant : Constant  Value=2.7
  Wind Speed measured at 2m height (u2) [m/s] : Subsystem
  Out1 : Outport
  wires:
  Wind Speed measured at 2m height (u2) [m/s]/1(u2) -> Out1/1
  [WindH] -> Wind Speed measured at 2m height (u2) [m/s]/2(z)
  Constant/1 -> Wind Speed measured at 2m height (u2) [m/s]/1(uz)

== system untitled_restored_from_autosave/Climate Model/ Historic Data/Humidity ==

== system untitled_restored_from_autosave/Climate Model/ Historic Data/Precipitation ==

== system untitled_restored_from_autosave/Climate Model/ Historic Data/Solar Radiation ==

== system untitled_restored_from_autosave/Climate Model/ Historic Data/Temperature [°C] ==

== system untitled_restored_from_autosave/Climate Model/ Historic Data/Wind Speed  ==

== system untitled_restored_from_autosave/Climate Model/AI Prediction/AI Solar Radiation [MJ//m^2//day] ==
  AI_Rs : Outport

== system untitled_restored_from_autosave/Climate Model/AI Prediction/Humidity ==

== system untitled_restored_from_autosave/Climate Model/AI Prediction/Precipitation ==

== system untitled_restored_from_autosave/Climate Model/AI Prediction/Temperature [°C] ==
  AI_T : Outport

== system untitled_restored_from_autosave/Climate Model/AI Prediction/Wind Speed [m//s] ==
  AI_Uz : Outport

== system untitled_restored_from_autosave/Estimated Soil Heat Capacity (UC Davis)/Bulk Density (Saxton and Rawls Function) [g//cm^3)/Normal Density (g//cm^3) ==
  Constant : Constant  Value=2.65
  Constant1 : Constant
  Product : Product
  Saturated Moisture θS : Subsystem
  Subtract : Sum  Inputs=+-
  Out1 : Outport
  wires:
  Product/1 -> Out1/1
  Constant/1 -> Product/2
  Subtract/1 -> Product/1
  Constant1/1 -> Subtract/1
  Saturated Moisture θS/1(Out1) -> Subtract/2

== system untitled_restored_from_autosave/Estimated Soil Heat Capacity (UC Davis)/Bulk Density (Saxton and Rawls Function) [g//cm^3)/Volum Fraction of Gravel (g//cm^3) ==
  In1 : Inport
  Constant : Constant  Value=2.65
  Constant1 : Constant
  Constant2 : Constant
  Divide : Product  Inputs=*/
  Divide1 : Product  Inputs=*/
  Product : Product
  Product1 : Product
  Subtract : Sum  Inputs=+-
  Subtract1 : Sum  Inputs=+-
  Out1 : Outport
  wires:
  In1/1 -> Divide/1
  [PGravel] -> Product1/1, Product/2
  Constant/1 -> Divide/2
  Divide/1 -> Subtract1/2, Product/1
  Product/1 -> Divide1/1
  Subtract/1 -> Divide1/2
  Constant1/1 -> Subtract/1
  Product1/1 -> Subtract/2
  Subtract1/1 -> Product1/2
  Constant2/1 -> Subtract1/1
  Divide1/1 -> Out1/1

== system untitled_restored_from_autosave/Normal Density (g//cm^3)/Saturated Moisture θS/θ(S-33) ==
  Constant : Constant  Value=0.636
  Constant1 : Constant  Value=0.107
  Product : Product
  Subtract : Sum  Inputs=++-
  θ(S-33)t : Subsystem
  Out1 : Outport
  wires:
  θ(S-33)t/1(Out1) -> Product/1, Subtract/1
  Product/1 -> Subtract/2
  Constant/1 -> Product/2
  Constant1/1 -> Subtract/3
  Subtract/1 -> Out1/1

== system untitled_restored_from_autosave/Plant Model/General Plant Database/Coarse Texture ==
  In1 : Inport
  2-D Lookup Table : Lookup_n-D  BreakpointsForDimension1=[0 1 2 3 4 5 6 7 8 9 10 11 12]  BreakpointsForDimension2=[1 2 3 4 5 6]  Table=|  InternalRulePriority=Speed  RndMeth=Simplest  InputSameDT=on
      | [1.15 1.15 1.15 1.15 1.15 1.15;
      | 1.15 1.15 1.15 1 0.7 0.35;
      | 1.15 1.15 1.05 0.7 0.5 0.25;
      | 1.15 1.15 0.875 0.575 0.4 0.2;
      | 1.15 1.075 0.775 0.425 0.35 0.175;
      | 1.15 1 0.65 0.4 0.28 0.15;
      | 1.13 0.94 0.575 0.35 0.25 0.125;
      | 1.1 0.86 0.52 0.3 0.21 0.1;
      | 1.075 0.8 0.45 0.27 0.18 0.08;
      | 1.05 0.73 0.41 0.23 0.16 0.07;
      | 1.01 0.675 0.375 0.21 0.14 0.06;
      | 0.975 0.63 0.34 0.19 0.13 0.055;
      | 0.925 0.6 0.31 0.175 0.12 0.05]
  Round : Rounding  Operator=round
  Out1 : Outport
  wires:
  [ET0] -> Round/1
  2-D Lookup Table/1 -> Out1/1
  In1/1 -> 2-D Lookup Table/2
  Round/1 -> 2-D Lookup Table/1

== system untitled_restored_from_autosave/Plant Model/General Plant Database/Fine and Medium Texture ==
  In1 : Inport
  2-D Lookup Table : Lookup_n-D  BreakpointsForDimension1=[0 1 2 3 4 5 6 7 8 9 10 11 12]  BreakpointsForDimension2=[1 2 3 4 5 6]  Table=|  InternalRulePriority=Speed  RndMeth=Simplest  InputSameDT=on
      | [1.15 1.15 1.15 1.15 1.15 1.15;
      | 1.15 1.15 1.15 1.15 1.15 0.65;
      | 1.15 1.15 1.15 1.125 0.85 0.45;
      | 1.15 1.15 1.1 0.87 0.7 0.38;
      | 1.15 1.15 1.025 0.7 0.6 0.325;
      | 1.15 1.125 0.95 0.65 0.5 0.275;
      | 1.15 1.1 0.875 0.6 0.45 0.225;
      | 1.15 1.06 0.81 0.54 0.4 0.2;
      | 1.15 1.025 0.73 0.48 0.35 0.175;
      | 1.14 0.98 0.675 0.43 0.3 0.15;
      | 1.125 0.94 0.63 0.39 0.275 0.125;
      | 1.1 0.9 0.59 0.35 0.25 0.11;
      | 1.08 0.85 0.55 0.31 0.225 0.1]
  Round : Rounding  Operator=round
  Out1 : Outport
  wires:
  2-D Lookup Table/1 -> Out1/1
  [ET0] -> Round/1
  In1/1 -> 2-D Lookup Table/2
  Round/1 -> 2-D Lookup Table/1

== system untitled_restored_from_autosave/Plant Model/General Plant Database/Subsystem ==
  In1 : Inport
  2-D Lookup Table : Lookup_n-D  BreakpointsForDimension1=[0 1 2 3 4 5 6 7 8 9 10 11 12]  BreakpointsForDimension2=[1 2 3 4 5 6]  Table=|  InternalRulePriority=Speed  RndMeth=Simplest  InputSameDT=on
      | [1.15 1.15 1.15 1.15 1.15 1.15; 
      | 1.15 1.15 1.15 1.15 0.9 0.5; 
      | 1.15 1.15 1 0.675 0.5 0.25;
      | 1.15 1.05 0.7 0.475 0.325 0.175;
      | 1.1 0.9 0.6 0.35 0.25 0.125;
      | 1.05 0.775 0.475 0.275 0.2 0.1;
      | 0.95 0.7 0.41 0.225 0.175 0.08;
      | 0.9 0.625 0.35 0.21 0.15 0.07;
      | 0.875 0.575 0.3 0.18 0.125 0.06;
      | 0.825 0.525 0.275 0.16 0.11 0.05;
      | 0.775 0.475 0.25 0.14 0.1 0.045;
      | 0.725 0.425 0.225 0.125 0.09 0.04;
      | 0.7 0.4 0.2 0.11 0.08 0.04]
  Round : Rounding  Operator=round
  Out1 : Outport
  wires:
  In1/1 -> 2-D Lookup Table/2
  2-D Lookup Table/1 -> Out1/1
  [ET0] -> Round/1
  Round/1 -> 2-D Lookup Table/1

== system untitled_restored_from_autosave/Reference Evapotraspiration (ET0) [mm//day]/Actual Vapor Pressure (ea) [kPa]/Derived from Dewpoint Temperature ==
  Saturation Vapor Pressure (eo) : Subsystem
  Out1 : Outport
  wires:
  [Tdew] -> Saturation Vapor Pressure (eo)/1(In1)
  Saturation Vapor Pressure (eo)/1(Out1) -> Out1/1

== system untitled_restored_from_autosave/Reference Evapotraspiration (ET0) [mm//day]/Actual Vapor Pressure (ea) [kPa]/Derived from Psychrometric Data ==
  Constant : Constant  Value=apsy
  Product : Product
  Product1 : Product
  Saturation Vapor Pressure (eo) : Subsystem
  Subtract : Sum  Inputs=+-
  Subtract1 : Sum  Inputs=+-
  Out1 : Outport
  wires:
  Subtract/1 -> Out1/1
  Saturation Vapor Pressure (eo)/1(Out1) -> Subtract/1
  [Twet] -> Subtract1/2, Saturation Vapor Pressure (eo)/1(In1)
  [Tdry] -> Subtract1/1
  Subtract1/1 -> Product/1
  Product/1 -> Subtract/2
  Product1/1 -> Product/2
  [P] -> Product1/2
  Constant/1 -> Product1/1

== system untitled_restored_from_autosave/Reference Evapotraspiration (ET0) [mm//day]/Actual Vapor Pressure (ea) [kPa]/Derived from RHmax & RHmin ==
  Add : Sum
  Constant : Constant  Value=100
  Constant1 : Constant  Value=2
  Constant2 : Constant  Value=100
  Divide : Product  Inputs=**/
  Divide1 : Product  Inputs=**/
  Divide2 : Product  Inputs=*/
  Saturation Vapor Pressure (eo) : Subsystem
  Saturation Vapor Pressure (eo)1 : Subsystem
  Out1 : Outport
  wires:
  Divide2/1 -> Out1/1
  [Tmin] -> Saturation Vapor Pressure (eo)/1(In1)
  Saturation Vapor Pressure (eo)/1(Out1) -> Divide/1
  [RHmax] -> Divide/2
  Constant/1 -> Divide/3
  Divide/1 -> Add/1
  Divide1/1 -> Add/2
  Add/1 -> Divide2/1
  Constant1/1 -> Divide2/2
  Constant2/1 -> Divide1/3
  [RHmin] -> Divide1/2
  [Tmax] -> Saturation Vapor Pressure (eo)1/1(In1)
  Saturation Vapor Pressure (eo)1/1(Out1) -> Divide1/1

== system untitled_restored_from_autosave/Reference Evapotraspiration (ET0) [mm//day]/Actual Vapor Pressure (ea) [kPa]/Derived from RHmax only ==
  Constant : Constant  Value=100
  Divide : Product  Inputs=**/
  Saturation Vapor Pressure (eo) : Subsystem
  Out1 : Outport
  wires:
  Constant/1 -> Divide/3
  [Tmin] -> Saturation Vapor Pressure (eo)/1(In1)
  [RHmax] -> Divide/2
  Saturation Vapor Pressure (eo)/1(Out1) -> Divide/1
  Divide/1 -> Out1/1

== system untitled_restored_from_autosave/Reference Evapotraspiration (ET0) [mm//day]/Actual Vapor Pressure (ea) [kPa]/Derived from RHmean only ==
  Add : Sum
  Constant : Constant  Value=2
  Constant1 : Constant  Value=100
  Divide : Product  Inputs=*/
  Divide1 : Product  Inputs=*/
  Product : Product
  Saturation Vapor Pressure (eo) : Subsystem
  Saturation Vapor Pressure (eo)1 : Subsystem
  Out1 : Outport
  wires:
  [Tmax] -> Saturation Vapor Pressure (eo)/1(In1)
  Saturation Vapor Pressure (eo)/1(Out1) -> Add/1
  Saturation Vapor Pressure (eo)1/1(Out1) -> Add/2
  [Tmin] -> Saturation Vapor Pressure (eo)1/1(In1)
  Add/1 -> Divide/1
  Constant/1 -> Divide/2
  Divide/1 -> Product/2
  [RHmean] -> Divide1/1
  Constant1/1 -> Divide1/2
  Divide1/1 -> Product/1
  Product/1 -> Out1/1

== system untitled_restored_from_autosave/Reference Evapotraspiration (ET0) [mm//day]/Mean Saturation Vapor Pressure (es) [kPa] /Saturation Vapor Pressure (eo) ==
  In1 : Inport
  Add : Sum
  Constant : Constant  Value=0.6108
  Constant1 : Constant  Value=17.27
  Constant2 : Constant  Value=237.3
  Divide : Product  Inputs=**/
  Math Function : Math  SaturateOnIntegerOverflow=on
  Product : Product
  Out1 : Outport
  wires:
  Product/1 -> Out1/1
  Constant1/1 -> Divide/1
  In1/1 -> Add/1, Divide/2
  Add/1 -> Divide/3
  Divide/1 -> Math Function/1
  Constant/1 -> Product/1
  Constant2/1 -> Add/2
  Math Function/1 -> Product/2

== system untitled_restored_from_autosave/Reference Evapotraspiration (ET0) [mm//day]/Mean Saturation Vapor Pressure (es) [kPa] /Saturation Vapor Pressure (eo) 2 ==
  In1 : Inport
  Add1 : Sum
  Constant3 : Constant  Value=0.6108
  Constant4 : Constant  Value=17.27
  Constant5 : Constant  Value=237.3
  Divide1 : Product  Inputs=**/
  Math Function1 : Math  SaturateOnIntegerOverflow=on
  Product1 : Product
  Out1 : Outport
  wires:
  Math Function1/1 -> Product1/2
  Constant4/1 -> Divide1/1
  Add1/1 -> Divide1/3
  Constant3/1 -> Product1/1
  Divide1/1 -> Math Function1/1
  In1/1 -> Divide1/2, Add1/1
  Product1/1 -> Out1/1
  Constant5/1 -> Add1/2

== system untitled_restored_from_autosave/Reference Evapotraspiration (ET0) [mm//day]/Psychrometric Constant (Y) [kPA//°C]/Latent Heat of Vaporization (l) [MJ//kg] ==
  "Latent Heat for an Air Temperature of about 20°C " : Constant  Value=2.45
  l : Outport
  wires:
  "Latent Heat for an Air Temperature of about 20°C "/1 -> l/1

== system untitled_restored_from_autosave/Reference Evapotraspiration (ET0) [mm//day]/Soil Heat Flux Density (G) [MJ//m^2//day]/Long Time Steps ==
  Divide : Product  Inputs=**/*
  Subtract : Sum  Inputs=+-
  Out1 : Outport
  wires:
  [cs] -> Divide/1
  [Tmean] -> Subtract/1
  [Tpast] -> Subtract/2
  Subtract/1 -> Divide/2
  [Tpast_t] -> Divide/3
  [Zr] -> Divide/4
  Divide/1 -> Out1/1

== system untitled_restored_from_autosave/Soil Data Calculation/Estimated Soil Heat Capacity (UC Davis)/Bulk Density (Saxton and Rawls Function) [g//cm^3) ==
  Add : Sum
  Constant : Constant
  Constant1 : Constant  Value=2.65
  Normal Density (g/cm^3) : Subsystem
  Product : Product
  Product1 : Product
  Subtract : Sum  Inputs=+-
  Volum Fraction of Gravel (g/cm^3) : Subsystem
  Out1 : Outport
  wires:
  Add/1 -> Out1/1
  Normal Density (g/cm^3)/1(Out1) -> Product/1, Volum Fraction of Gravel (g/cm^3)/1(In1)
  Subtract/1 -> Product/2
  Product/1 -> Add/1
  Constant/1 -> Subtract/1
  Product1/1 -> Add/2
  Constant1/1 -> Product1/2
  Volum Fraction of Gravel (g/cm^3)/1(Out1) -> Subtract/2, Product1/1

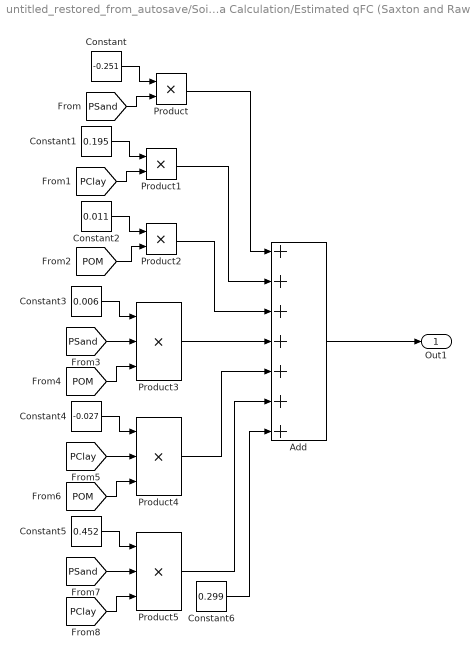
== system untitled_restored_from_autosave/Soil Data Calculation/Estimated qFC (Saxton and Rawls Function)/θ33t ==
  Add : Sum  Inputs=+++++++
  Constant : Constant  Value=-0.251
  Constant1 : Constant  Value=0.195
  Constant2 : Constant  Value=0.011
  Constant3 : Constant  Value=0.006
  Constant4 : Constant  Value=-0.027
  Constant5 : Constant  Value=0.452
  Constant6 : Constant  Value=0.299
  Product : Product
  Product1 : Product
  Product2 : Product
  Product3 : Product  Inputs=3
  Product4 : Product  Inputs=3
  Product5 : Product  Inputs=3
  Out1 : Outport
  wires:
  [PClay] -> Product5/3
  [PClay] -> Product1/2
  Constant4/1 -> Product4/1
  Product1/1 -> Add/2
  Constant3/1 -> Product3/1
  Product5/1 -> Add/6
  [PClay] -> Product4/2
  Product4/1 -> Add/5
  Constant6/1 -> Add/7
  Constant5/1 -> Product5/1
  [PSand] -> Product5/2
  Product/1 -> Add/1
  [PSand] -> Product/2
  Product2/1 -> Add/3
  Constant2/1 -> Product2/1
  Constant1/1 -> Product1/1
  Product3/1 -> Add/4
  Constant/1 -> Product/1
  [POM] -> Product2/2
  [PSand] -> Product3/2
  [POM] -> Product4/3
  [POM] -> Product3/3
  Add/1 -> Out1/1

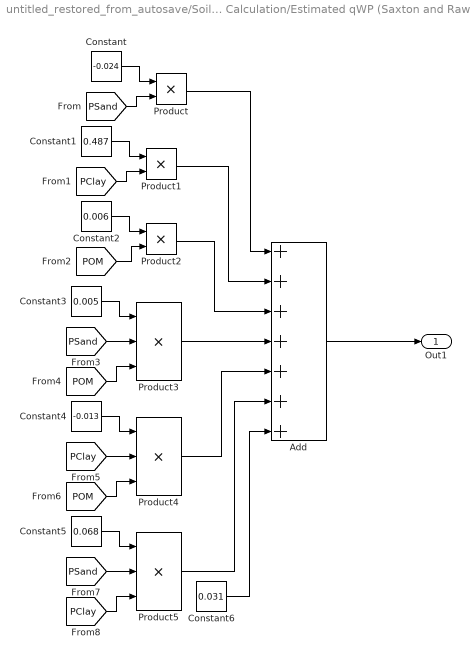
== system untitled_restored_from_autosave/Soil Data Calculation/Estimated qWP (Saxton and Rawls Function)/θ1500t ==
  Add : Sum  Inputs=+++++++
  Constant : Constant  Value=-0.024
  Constant1 : Constant  Value=0.487
  Constant2 : Constant  Value=0.006
  Constant3 : Constant  Value=0.005
  Constant4 : Constant  Value=-0.013
  Constant5 : Constant  Value=0.068
  Constant6 : Constant  Value=0.031
  Product : Product
  Product1 : Product
  Product2 : Product
  Product3 : Product  Inputs=3
  Product4 : Product  Inputs=3
  Product5 : Product  Inputs=3
  Out1 : Outport
  wires:
  [PClay] -> Product5/3
  [PClay] -> Product1/2
  Constant4/1 -> Product4/1
  Product1/1 -> Add/2
  Constant3/1 -> Product3/1
  Product5/1 -> Add/6
  [PClay] -> Product4/2
  Product4/1 -> Add/5
  Constant6/1 -> Add/7
  Constant5/1 -> Product5/1
  [PSand] -> Product5/2
  Product/1 -> Add/1
  [PSand] -> Product/2
  Product2/1 -> Add/3
  Constant2/1 -> Product2/1
  Constant1/1 -> Product1/1
  Product3/1 -> Add/4
  Constant/1 -> Product/1
  [POM] -> Product2/2
  [PSand] -> Product3/2
  [POM] -> Product4/3
  [POM] -> Product3/3
  Add/1 -> Out1/1

== system untitled_restored_from_autosave/Bulk Density (Saxton and Rawls Function) [g//cm^3)/Normal Density (g//cm^3)/Saturated Moisture θS/θ(S-33) ==
  Constant : Constant  Value=0.636
  Constant1 : Constant  Value=0.107
  Product : Product
  Subtract : Sum  Inputs=++-
  θ(S-33)t : Subsystem
  Out1 : Outport
  wires:
  θ(S-33)t/1(Out1) -> Product/1, Subtract/1
  Product/1 -> Subtract/2
  Constant/1 -> Product/2
  Constant1/1 -> Subtract/3
  Subtract/1 -> Out1/1

== system untitled_restored_from_autosave/Climate Model/ Final Calculation for Data/Daily Temperature [°C]/Mean Air Temperature at 2m height (Tmean) [°C] ==
  In1 : Inport
  Out1 : Outport
  wires:
  In1/1 -> Out1/1

== system untitled_restored_from_autosave/Climate Model/ Final Calculation for Data/Net Radiation at the Crop Surface (Rn) [MJ//m^2//day]/Clear-Sky Solar Radiation (Rso) [MJ//m^2//day] ==
  Add : Sum
  Constant : Constant  Value=0.75
  Constant1 : Constant  Value=0.00002
  Product : Product
  Product1 : Product
  Rso : Outport
  wires:
  Product/1 -> Rso/1
  [Ra] -> Product/2
  Add/1 -> Product/1
  Constant/1 -> Add/1
  Product1/1 -> Add/2
  [Altitude] -> Product1/2
  Constant1/1 -> Product1/1

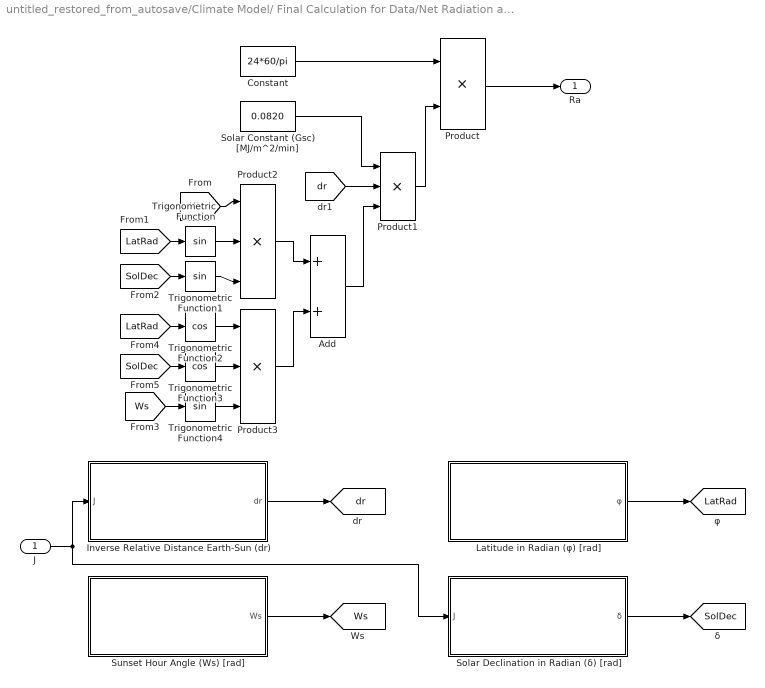
== system untitled_restored_from_autosave/Climate Model/ Final Calculation for Data/Net Radiation at the Crop Surface (Rn) [MJ//m^2//day]/Extraterrestrial Radiation (Ra) [MJ//m^2//day] ==
  J : Inport
  Add : Sum
  Constant : Constant  Value=24*60/pi
  Inverse Relative Distance Earth-Sun (dr) : Subsystem
  Latitude in Radian (φ) [rad] : Subsystem
  Product : Product
  Product1 : Product  Inputs=3
  Product2 : Product  Inputs=3
  Product3 : Product  Inputs=3
  Solar Constant (Gsc) [MJ/m^2/min] : Constant  Value=0.0820
  Solar Declination in Radian (δ) [rad] : Subsystem
  Sunset Hour Angle (Ws) [rad] : Subsystem
  Trigonometric Function : Trigonometry
  Trigonometric Function1 : Trigonometry
  Trigonometric Function2 : Trigonometry  Operator=cos
  Trigonometric Function3 : Trigonometry  Operator=cos
  Trigonometric Function4 : Trigonometry
  Ra : Outport
  tag scope: LatRad=global, SolDec=global, Ws=global, dr=global
  wires:
  Constant/1 -> Product/1
  Product/1 -> Ra/1
  Product1/1 -> Product/2
  Solar Constant (Gsc) [MJ/m^2/min]/1 -> Product1/1
  Latitude in Radian (φ) [rad]/1(φ) -> [LatRad]
  Solar Declination in Radian (δ) [rad]/1(δ) -> [SolDec]
  Sunset Hour Angle (Ws) [rad]/1(Ws) -> [Ws]
  Inverse Relative Distance Earth-Sun (dr)/1(dr) -> [dr]
  [dr] -> Product1/2
  Trigonometric Function/1 -> Product2/2
  Trigonometric Function1/1 -> Product2/3
  [Ws] -> Product2/1
  [LatRad] -> Trigonometric Function/1
  [SolDec] -> Trigonometric Function1/1
  Product2/1 -> Add/1
  Add/1 -> Product1/3
  [SolDec] -> Trigonometric Function3/1
  [LatRad] -> Trigonometric Function2/1
  Product3/1 -> Add/2
  Trigonometric Function2/1 -> Product3/1
  Trigonometric Function3/1 -> Product3/2
  Trigonometric Function4/1 -> Product3/3
  [Ws] -> Trigonometric Function4/1
  J/1 -> Solar Declination in Radian (δ) [rad]/1(J), Inverse Relative Distance Earth-Sun (dr)/1(J)
